simulink model "practica_1_diagrama_func"  (R2024a)
settings: Solver=VariableStepAuto  StartTime=0.0  StopTime=10.0  RelTol=1e-3
values from neighbouring files (symbols this model uses):
  g = 9.81    [Practica 1_1.m]    (also in Practica1_valores.m)
  l1 = 0.3    [Practica 1_1.m]    (also in Practica1_valores.m)
  l2 = 0.25    [Practica 1_1.m]    (also in Practica1_valores.m)
  m1 = 0.2    [Practica 1_1.m]    (also in Practica1_valores.m)
  m2 = 0.1    [Practica 1_1.m]    (also in Practica1_valores.m)

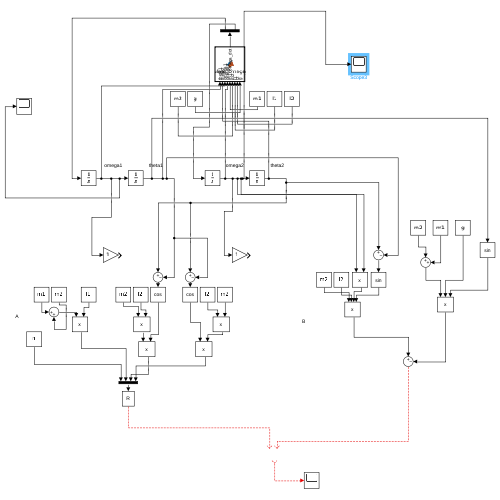
[thumbnail: Simulink's stored preview of the top-level diagram]
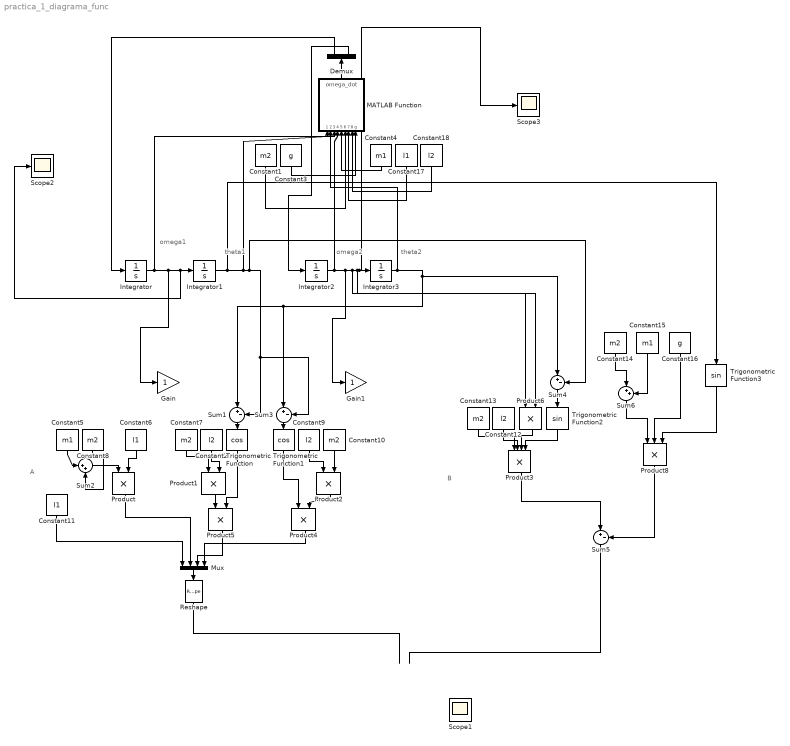
== system practica_1_diagrama_func ==
  note: B
  note: A
  note: theta2
  note: omega2
  note: theta1
  note: omega1
  Constant{1,7..8,10,13..14} (6 alike) : Constant  Value=m2
  Constant11 : Constant  Value=l1
  Constant{2,9,12,18} (4 alike) : Constant  Value=l2
  Constant15 : Constant  Value=m1
  Constant16 : Constant  Value=g
  Constant17 : Constant  Value=l1
  Constant3 : Constant  Value=g
  Constant4 : Constant  Value=m1
  Constant5 : Constant  Value=m1
  Constant6 : Constant  Value=l1
  Demux : Demux  Outputs=2
  Gain : Gain
  Gain1 : Gain
  Integrator : Integrator
  Integrator1 : Integrator
  Integrator2 : Integrator
  Integrator3 : Integrator  InitialCondition=deg2rad(35)
  MATLAB Function : MATLAB Function  TreatAsAtomicUnit=on
  Mux : Mux
  Product{,1..2,4..6} (6 alike) : Product
  Product3 : Product  Inputs=4
  Product8 : Product  Inputs=3
  Reshape : Reshape  OutputDimensionality=Customize  OutputDimensions=[2,2]
  Scope1 : Scope
  Scope2 : Scope
  Scope3 : Scope
  Sum{1,3..5} (4 alike) : Sum  Inputs=|+-
  Sum2 : Sum  Inputs=|++
  Sum6 : Sum  Inputs=|++
  Trigonometric Function : Trigonometry  Operator=cos
  Trigonometric Function1 : Trigonometry  Operator=cos
  Trigonometric Function2 : Trigonometry
  Trigonometric Function3 : Trigonometry
  wires:
  Integrator/1 -> Gain/1, Scope2/1, Integrator1/1, MATLAB Function/3(omega1)
  Integrator2/1 -> MATLAB Function/4(omega2), Scope3/1, Integrator3/1, Product6/2, Product6/1, Gain1/1
  Constant5/1 -> Sum2/1
  Constant6/1 -> Product/2
  Constant7/1 -> Product1/1
  Constant2/1 -> Product1/2
  Trigonometric Function/1 -> Product5/2
  Sum1/1 -> Trigonometric Function/1
  Integrator3/1 -> Sum4/1, Sum3/1, Sum1/1, MATLAB Function/2(theta2)
  Integrator1/1 -> Trigonometric Function3/1, Sum3/2, Sum1/2, Sum4/2, MATLAB Function/1(theta1)
  Constant8/1 -> Sum2/2
  Sum2/1 -> Product/1
  Sum3/1 -> Trigonometric Function1/1
  Trigonometric Function1/1 -> Product4/1
  Constant9/1 -> Product2/1
  Constant10/1 -> Product2/2
  Product2/1 -> Product4/2
  Constant11/1 -> Mux/1
  Product/1 -> Mux/2
  Product5/1 -> Mux/3
  Product1/1 -> Product5/1
  Product4/1 -> Mux/4
  Mux/1 -> Reshape/1
  Sum4/1 -> Trigonometric Function2/1
  Constant13/1 -> Product3/1
  Constant12/1 -> Product3/2
  Product6/1 -> Product3/3
  Trigonometric Function2/1 -> Product3/4
  Product3/1 -> Sum5/1
  Constant14/1 -> Sum6/1
  Constant15/1 -> Sum6/2
  Sum6/1 -> Product8/1
  Constant16/1 -> Product8/2
  Trigonometric Function3/1 -> Product8/3
  Product8/1 -> Sum5/2
  Constant1/1 -> MATLAB Function/6(m2)
  Constant3/1 -> MATLAB Function/9(g)
  Constant4/1 -> MATLAB Function/5(m1)
  Constant17/1 -> MATLAB Function/7(l1)
  Constant18/1 -> MATLAB Function/8(l2)
  Reshape/1 -> ?
  Sum5/1 -> ?
  ? -> Scope1/1
  MATLAB Function/1(omega_dot) -> Demux/1
  Demux/1 -> Integrator/1
  Demux/2 -> Integrator2/1

== matlab function practica_1_diagrama_func/MATLAB Function ==
  data: theta1 input; omega_dot output; theta2 input; omega1 input; omega2 input; m1 input; m2 input; l1 input; l2 input; g input
function omega_dot = calculate_omega_dot(theta1, theta2, omega1, omega2, m1, m2, l1, l2, g)
    omega_dot = zeros(2,1) 
    % Calcular elementos de la matriz A
    A11 = (m1 + m2) * l1;
    A12 = m2 * l2 * cos(theta2 - theta1);
    A21 = A12;  % Simetría
    A22 = l1;
    
    % Definir matriz A de tamaño 2x2
    A = [A11, A12; A21, A22];

    % Calcular elementos del vector B
    B1 = -(m2 * l2 * omega2^2 * sin(theta2 - theta1)) - (m1 + m2) * g * sin(theta1);
    B2 = -(l1 * omega1^2 * sin(theta2 - theta1)) - g * sin(theta2);
    
    % Definir vector B de tamaño 2x1
    B = [B1; B2];

    % Resolver sistema lineal A * omega_dot = B
    omega_dot = A \ B;
end
